simulink model "Mars_Rover_Params"  (R2022b)
settings: Solver=ode8  StartTime=0.0  StopTime=100  FixedStep=0.1  RelTol=1e-3
settings Model: Creator=basti  LastModifiedBy=basti
settings DataIOCC: SaveFormat=Array  ReturnWorkspaceOutputs=off
settings DebuggingCC: UnconnectedInputMsg=warning  UnconnectedOutputMsg=warning  UnconnectedLineMsg=warning
settings ModelReferenceCC: EnableRefExpFcnMdlSchedulingChecks=on
settings RTWCC: DLArmComputeVersion=19.05

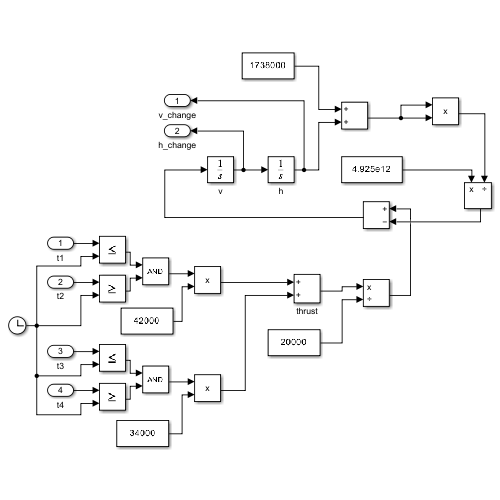
[thumbnail: Simulink's stored preview of the top-level diagram]
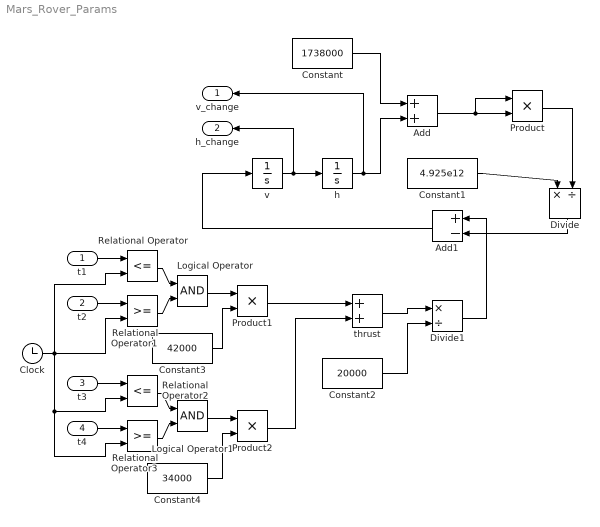
== system Mars_Rover_Params ==
  t1 : Inport
  t2 : Inport  Port=2
  t3 : Inport  Port=3
  t4 : Inport  Port=4
  Add : Sum
  Add1 : Sum  Inputs=+-
  Clock : Clock
  Constant : Constant  Value=1738000
  Constant1 : Constant  Value=4.925e12
  Constant2 : Constant  Value=20000
  Constant3 : Constant  Value=42000
  Constant4 : Constant  Value=34000
  Divide : Product  Inputs=*/
  Divide1 : Product  Inputs=*/
  Logical Operator : Logic  AllPortsSameDT=off  OutDataTypeStr=boolean
  Logical Operator1 : Logic  AllPortsSameDT=off  OutDataTypeStr=boolean
  Product : Product
  Product1 : Product
  Product2 : Product
  Relational Operator : RelationalOperator  Operator=<=  OutDataTypeStr=boolean  RndMeth=Simplest  InputSameDT=off
  Relational Operator1 : RelationalOperator  OutDataTypeStr=boolean  RndMeth=Simplest  InputSameDT=off
  Relational Operator2 : RelationalOperator  Operator=<=  OutDataTypeStr=boolean  RndMeth=Simplest  InputSameDT=off
  Relational Operator3 : RelationalOperator  OutDataTypeStr=boolean  RndMeth=Simplest  InputSameDT=off
  h : Integrator  InitialCondition=1000
  thrust : Sum
  v : Integrator  InitialCondition=-10
  v_change : Outport
  h_change : Outport  Port=2
  wires:
  v/1 -> h_change/1, h/1
  h/1 -> v_change/1, Add/2
  Constant/1 -> Add/1
  Add/1 -> Product/1, Product/2
  Product/1 -> Divide/2
  Constant1/1 -> Divide/1
  Constant2/1 -> Divide1/2
  thrust/1 -> Divide1/1
  Divide1/1 -> Add1/1
  Divide/1 -> Add1/2
  Add1/1 -> v/1
  t1/1 -> Relational Operator/1
  Clock/1 -> Relational Operator3/2, Relational Operator2/2, Relational Operator1/2, Relational Operator/2
  t2/1 -> Relational Operator1/1
  Relational Operator/1 -> Logical Operator/1
  Relational Operator1/1 -> Logical Operator/2
  Logical Operator/1 -> Product1/1
  Product1/1 -> thrust/1
  t3/1 -> Relational Operator2/1
  t4/1 -> Relational Operator3/1
  Relational Operator2/1 -> Logical Operator1/1
  Relational Operator3/1 -> Logical Operator1/2
  Constant3/1 -> Product1/2
  Logical Operator1/1 -> Product2/1
  Constant4/1 -> Product2/2
  Product2/1 -> thrust/2
